simulink model "controller_unst"  (R2015a)
settings: Solver=FixedStepDiscrete  StartTime=0.0  StopTime=inf  FixedStep=0.01  RelTol=1e-3
libraries: PoliArd x8, simulink x2
settings Model: ExtModeTrigDuration=2  Creator=user  LastModifiedBy=lelli
settings OptimizationCC: OptimizeModelRefInitCode=on  LifeSpan=1
settings DebuggingCC: UnderspecifiedInitializationDetection=Classic  MergeDetectMultiDrivingBlocksExec=none
settings HardwareCC: ProdLargestAtomicInteger=Long  ProdLargestAtomicFloat=Double  ProdEndianess=LittleEndian  ProdHWDeviceType=ARM Compatible->ARM Cortex
settings RTWCC: SystemTargetFile=realtime.tlc  GenerateMakefile=off  TemplateMakefile=realtime.tmf  Description=Run on Target Hardware  RTWVerbose=off
settings ERTTargetCC: CombineOutputUpdateFcns=off  ExtModeTransport=3  ExtModeMexFile=ext_serial_win32_comm_rtt  ExtModeMexArgs=0 1 9600  ERTSrcFileBannerTemplate=realtime_code_template.cgt  ERTHdrFileBannerTemplate=realtime_code_template.cgt  ERTDataSrcFileTemplate=realtime_code_template.cgt  ERTDataHdrFileTemplate=realtime_code_template.cgt  ERTCustomFileTemplate=realtime_file_process.tlc

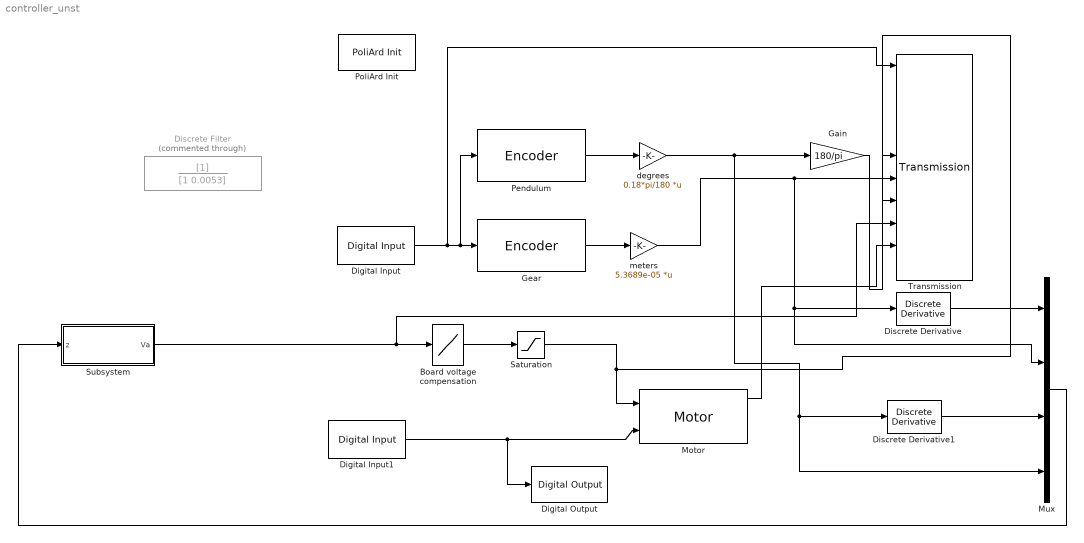
== system controller_unst ==
  Board voltage compensation : Lookup_n-D  NumberOfTableDimensions=1  BreakpointsForDimension1=[-11.90 -10.89 -10.05 -8.92 -7.80 -6.96 -5.98 -5.01 -3.98 -2.95 -2.02 -1.94 -1.85 -1.75 -1.56 -1.47 -1.37 -1.28 -1.18 -1.08 -0.98 -0.87 -0.77 -0.63 -0.53 -0.35 -0.06 0.0 0.08 0.34 0.51 0.63 0.75 0.88 0.99 1.00 1.19 1.39 1.48 1.58 1.67 1.77 1.86 1.96 2.04 3.07 4.00 5.07 5.96 6.98 7.98 9.03 10.02 10.99 11.93]  Table=[-12 -10.90 -10.11 -9.00 -7.84 -6.96 -6.0 -5.02 -4.01 -2.94 -2.0 -1.89 -1.79 -1.70 -1.59 -1.49 -1.39 -1.30 -1.20 -1.09 -0.99 -0.89 -0.80 -0.71 -0.59 -0.50 -0.40 0 0.42 0.52 0.59 0.71 0.80 0.91 1.00 1.11 1.21 1.35 1.44 1.52 1.62 1.70 1.81 1.90 2.00 3.02 4.01 5.06 5.97 6.97 7.97 9.05 10.03 11.01 12.00]  InternalRulePriority=Speed  RndMeth=Simplest  InputSameDT=on
  Digital Input : PoliArd/Digital Input  DI_pin=2  DIsample=-1
  Digital Input1 : PoliArd/Digital Input  DI_pin=3  DIsample=-1
  Digital Output : PoliArd/Digital Output  DO_pin=1
  Discrete Derivative : simulink/Discrete/Discrete Derivative  gainval=1.0  ICPrevScaledInput=0.0  InputProcessing=Inherited  OutMin=[]  OutMax=[]  OutDataType=fixdt(1, 16)  OutScaling=2^-10  DoSatur=off
  Discrete Derivative1 : simulink/Discrete/Discrete Derivative  gainval=1.0  ICPrevScaledInput=0.0  InputProcessing=Inherited  OutMin=[]  OutMax=[]  OutDataType=fixdt(1, 16)  OutScaling=2^-10  DoSatur=off
  Discrete Filter : DiscreteFilter  Commented=through  Denominator=[1 0.0053]
  Gain : Gain  Gain=180/pi
  Gear : PoliArd/Encoder  EncoderID=3  dt_enc=-1
  Motor : PoliArd/Motor  MotorID=1  DC_bus_mask=12  dt_mot=-1
  Mux : Mux
  "Pendulum " : PoliArd/Encoder  EncoderID=1  dt_enc=-1
  PoliArd Init : PoliArd/PoliArd Init
  Saturation : Saturate  UpperLimit=12  LowerLimit=-12
  Subsystem : Subsystem
  Transmission : PoliArd/Transmission  sample_freq=100  sig_to_send=6
  degrees : Gain  Gain=0.18*pi/180  Multiplication=Matrix(K*u)  ParamDataTypeStr=double
  meters : Gain  Gain=5.3689e-05  Multiplication=Matrix(K*u)  ParamDataTypeStr=double
  wires:
  "Pendulum "/1 -> degrees/1
  Gear/1 -> meters/1
  Digital Input1/1 -> Digital Output/1, Motor/2
  Motor/1 -> Transmission/9
  Digital Input/1 -> Transmission/1, "Pendulum "/1, Gear/1
  Mux/1 -> Subsystem/1(z)
  meters/1 -> Transmission/6, Discrete Derivative/1, Mux/2
  Saturation/1 -> Motor/1, Transmission/7
  Board voltage compensation/1 -> Saturation/1
  Discrete Derivative/1 -> Mux/1
  Discrete Derivative1/1 -> Mux/3
  degrees/1 -> Gain/1, Discrete Derivative1/1, Mux/4
  Subsystem/1(Va) -> Transmission/8, Board voltage compensation/1
  Gain/1 -> Transmission/5

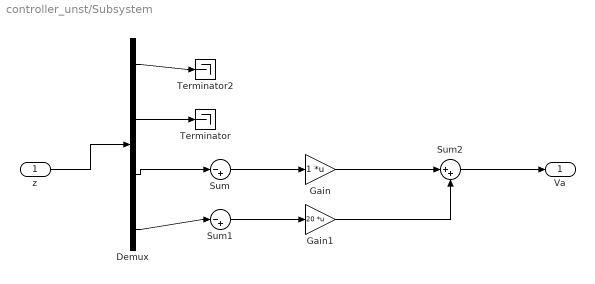
== system controller_unst/Subsystem ==
  z : Inport
  Demux : Demux
  Gain : Gain  Multiplication=Matrix(K*u)
  Gain1 : Gain  Gain=20  Multiplication=Matrix(K*u)
  Sum : Sum  Inputs=|-+
  Sum1 : Sum  Inputs=|-+
  Sum2 : Sum  Inputs=|++
  Terminator : Terminator
  Terminator2 : Terminator
  Va : Outport
  wires:
  z/1 -> Demux/1
  Demux/4 -> Sum1/1
  Sum1/1 -> Gain1/1
  Demux/3 -> Sum/1
  Gain1/1 -> Sum2/2
  Gain/1 -> Sum2/1
  Sum/1 -> Gain/1
  Sum2/1 -> Va/1
  Demux/1 -> Terminator2/1
  Demux/2 -> Terminator/1
